simulink subsystem "ApplicationMotorSwapLowPrio"  (R2024b)
settings: Solver=VariableStepAuto  StartTime=0.0  StopTime=10.0  RelTol=1e-3
undefined symbols (not defined in the file or in its folder): inverter, pmsm
libraries: simulink x1, slpidlib x1
settings Model: Creator=The MathWorks, Inc.  LastModifiedBy=snarayan
settings RTWCC: GPUComputeCapability=3.5

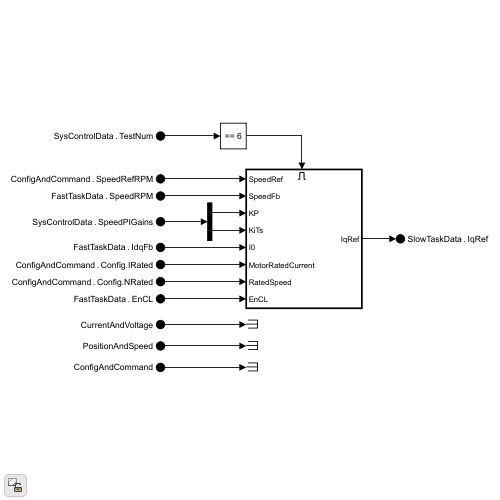
[thumbnail: Simulink's stored preview of the top-level diagram]
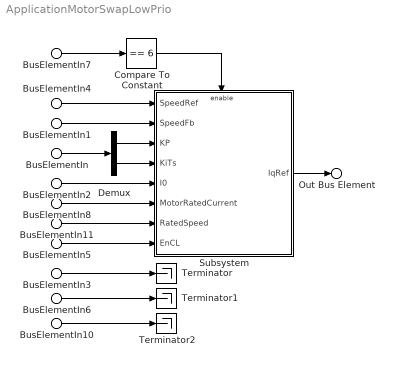
== system ApplicationMotorSwapLowPrio ==
  BusElementIn10 : Inport  PortName=ConfigAndCommand
  BusElementIn4 : Inport  PortName=ConfigAndCommand  Element=SpeedRefRPM
  BusElementIn8 : Inport  PortName=ConfigAndCommand  Element=Config.IRated
  BusElementIn11 : Inport  PortName=ConfigAndCommand  Element=Config.NRated
  BusElementIn3 : Inport  Port=2  PortName=CurrentAndVoltage
  BusElementIn6 : Inport  Port=3  PortName=PositionAndSpeed
  BusElementIn2 : Inport  Port=4  PortName=FastTaskData  Element=IdqFb
  BusElementIn1 : Inport  Port=4  PortName=FastTaskData  Element=SpeedRPM
  BusElementIn5 : Inport  Port=4  PortName=FastTaskData  Element=EnCL
  BusElementIn7 : Inport  Port=5  PortName=SysControlData  Element=TestNum
  BusElementIn : Inport  Port=5  PortName=SysControlData  Element=SpeedPIGains
  Compare To Constant : simulink/Logic and Bit Operations/Compare To Constant  relop===  const=6  OutDataTypeStr=boolean
  Demux : Demux  Outputs=2
  Subsystem : Subsystem
  Terminator : Terminator
  Terminator1 : Terminator
  Terminator2 : Terminator
  Out Bus Element : Outport  PortName=SlowTaskData  Element=IqRef
  wires:
  BusElementIn4/1 -> Subsystem/1(SpeedRef)
  BusElementIn1/1 -> Subsystem/2(SpeedFb)
  BusElementIn2/1 -> Subsystem/5(I0)
  BusElementIn3/1 -> Terminator/1
  Subsystem/1(IqRef) -> Out Bus Element/1
  BusElementIn7/1 -> Compare To Constant/1
  Compare To Constant/1 -> Subsystem/Enable
  BusElementIn6/1 -> Terminator1/1
  BusElementIn10/1 -> Terminator2/1
  BusElementIn8/1 -> Subsystem/6(MotorRatedCurrent)
  BusElementIn11/1 -> Subsystem/7(RatedSpeed)
  Demux/1 -> Subsystem/3(KP)
  Demux/2 -> Subsystem/4(KiTs)
  BusElementIn/1 -> Demux/1
  BusElementIn5/1 -> Subsystem/8(EnCL)

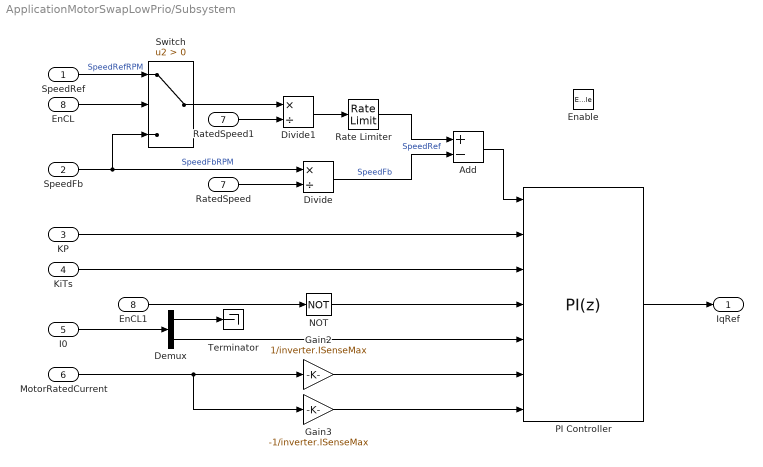
== system ApplicationMotorSwapLowPrio/Subsystem ==
  SpeedRef : Inport
  SpeedFb : Inport  Port=2
  KP : Inport  Port=3
  KiTs : Inport  Port=4
  I0 : Inport  Port=5
  MotorRatedCurrent : Inport  Port=6
  RatedSpeed : Inport  Port=7
  EnCL : Inport  Port=8
  Enable : EnablePort
  Add : Sum  Inputs=+-
  Demux : Demux  Outputs=2
  Divide : Product  Inputs=*/
  Divide1 : Product  Inputs=*/
  EnCL1 : InportShadow  Port=8
  Gain2 : Gain  Gain=1/inverter.ISenseMax  RndMeth=Simplest  OutDataTypeStr=Inherit: Same as input
  Gain3 : Gain  Gain=-1/inverter.ISenseMax  RndMeth=Simplest  OutDataTypeStr=Inherit: Same as input
  NOT : Logic  Operator=NOT  IconShape=distinctive  AllPortsSameDT=off  OutDataTypeStr=boolean
  PI Controller : slpidlib/PID Controller  Controller=PI  Form=Parallel  TimeDomain=Discrete-time  UseExternalTs=off  SampleTime=-1  IntegratorMethod=Forward Euler  FilterMethod=Forward Euler  ControllerParametersSource=external  P=1  I=1  UseKiTs=on  D=0  UseExternalDerivativeSource=off  N=100  UseFilter=on  TunerSelectOption=Transfer Function Based (PID Tuner App)  InitialConditionSource=external  InitialConditionForIntegrator=0  InitialConditionForFilter=0  DifferentiatorICPrevScaledInput=0  ExternalReset=level  TrackingMode=off  Kt=1  LimitOutput=on  SatLimitsSource=external  UpperSaturationLimit=pmsm.I_rated  LowerSaturationLimit=-pmsm.I_rated  LinearizeAsGain=on  AntiWindupMode=clamping  Kb=1  LimitIntegrator=off  UpperIntegratorSaturationLimit=inf  LowerIntegratorSaturationLimit=-inf  RndMeth=Simplest  POutMin=[]  POutMax=[]  IOutMin=[]  IOutMax=[]  DOutMin=[]  DOutMax=[]  NOutMin=[]  NOutMax=[]  SumOutMin=[]  SumOutMax=[]  SaturationOutDataTypeStr=Inherit: Inherit via back propagation  SaturationOutMin=[]  SaturationOutMax=[]  PParamMin=[]  PParamMax=[]  IParamMin=[]  IParamMax=[]  DParamMin=[]  DParamMax=[]  NParamMin=[]  NParamMax=[]  KbParamMin=[]  KbParamMax=[]  KtParamMin=[]  KtParamMax=[]  KbOutMin=[]  KbOutMax=[]  KtOutMin=[]  KtOutMax=[]  IntegratorOutMin=[]  IntegratorOutMax=[]  FilterOutMin=[]  FilterOutMax=[]  SumI1OutMin=[]  SumI1OutMax=[]  SumI2OutMin=[]  SumI2OutMax=[]  SumI3OutMin=[]  SumI3OutMax=[]  SumI4OutMin=[]  SumI4OutMax=[]  SumDOutMin=[]  SumDOutMax=[]  DifferentiatorOutMin=[]  DifferentiatorOutMax=[]  FilterDiffOutCoefMin=[]  FilterDiffOutCoefMax=[]  ReciprocalOutMin=[]  ReciprocalOutMax=[]  SumDenOutMin=[]  SumDenOutMax=[]  SumNumOutMin=[]  SumNumOutMax=[]  DivideOutMin=[]  DivideOutMax=[]  UdiffTsProdOutMin=[]  UdiffTsProdOutMax=[]  NTsProdOutMin=[]  NTsProdOutMax=[]  UintegralTsProdOutMin=[]  UintegralTsProdOutMax=[]  UngainTsProdOutMin=[]  UngainTsProdOutMax=[]  ClampingZeroOutDataTypeStr=Inherit: Inherit via back propagation  ClampingZeroOutMin=[]  ClampingZeroOutMax=[]  FilterDenConstantOutDataTypeStr=Inherit: Inherit via back propagation  FilterDenConstantOutMin=[]  FilterDenConstantOutMax=[]  PCopyOutDataTypeStr=Inherit: Inherit via back propagation  PCopyOutMin=[]  PCopyOutMax=[]  NCopyOutDataTypeStr=Inherit: Inherit via back propagation  NCopyOutMin=[]  NCopyOutMax=[]  IntegratorContinuousStateAttributes=''  IntegratorStateMustResolveToSignalObject=off  IntegratorRTWStateStorageClass=Auto  FilterContinuousStateAttributes=''  FilterStateMustResolveToSignalObject=off  FilterRTWStateStorageClass=Auto  ParallelPVariant=ExternalParameters  IdealPVariant=Disabled  IVariant=ExternalParameters  DVariant=Disabled  IntegratorVariant=Discrete  SatVariant=External  AWVariant=DiscClampingParallel  PCopyVariant=Disabled  TRVariant=Disabled  FdbkBlocksVariant=Forward  IdealPFdbkVariant=Disabled  SatFdbkVariant=Disabled  DerivativeFilterVariant=Disabled  NVariant=Disabled  NCopyVariant=Disabled_SignalSpec  FilterICVariant=Disabled  IntegratorICVariant=ExternalICs  ExternalResetVariant=ExternalReset  TRSumVariant=Passthrough  SumFdbkVariant=Disabled  SumVariant=Sum_PI  TsampFilterVariant=InternalTs  TsampNgainVariant=Passthrough  TsampIntegralVariant=Disabled_SignalSpec  ExternalSaturationOutDataTypeStr=Inherit: Same as second input  DerivativeSourceVariant=Disabled  PreIntVariant=InternalPreInt
  Rate Limiter : RateLimiter  RisingSlewLimit=0.5  FallingSlewLimit=-0.5  SampleTimeMode=inherited
  RatedSpeed1 : InportShadow  Port=7
  Switch : Switch  Criteria=u2 > Threshold  SaturateOnIntegerOverflow=off  InputSameDT=off
  Terminator : Terminator
  IqRef : Outport
  wires:
  PI Controller/1 -> IqRef/1
  RatedSpeed1/1 -> Divide1/2
  Divide1/1 -> Rate Limiter/1
  Rate Limiter/1 -> Add/1  "SpeedRef"
  Divide/1 -> Add/2  "SpeedFb"
  SpeedFb/1 -> Switch/3, Divide/1  "SpeedFbRPM"
  RatedSpeed/1 -> Divide/2
  Demux/2 -> PI Controller/5
  KP/1 -> PI Controller/2
  Demux/1 -> Terminator/1
  EnCL/1 -> Switch/2
  EnCL1/1 -> NOT/1
  SpeedRef/1 -> Switch/1  "SpeedRefRPM"
  MotorRatedCurrent/1 -> Gain2/1, Gain3/1
  KiTs/1 -> PI Controller/3
  Switch/1 -> Divide1/1
  Add/1 -> PI Controller/1
  Gain3/1 -> PI Controller/7
  Gain2/1 -> PI Controller/6
  I0/1 -> Demux/1
  NOT/1 -> PI Controller/4
